simulink model "schemaABlocchi_2023b"  (R2023b)
settings: Solver=ode45  StartTime=0.0  StopTime=12  MaxStep=1e-3  RelTol=1e-3  EnableMultiTasking=on
PreLoadFcn:
  | clear %%clear workspace
  | 
  | %--------------------
  | %SYSTEM'S PARAMETERS [parametri del sistema]:
  | %--------------------
  | 
  | M = 0.5         %cart mass [massa del carrello]
  | m = 0.1         %sphere mass [massa estremità del asta]
  | g = 9,80665     %gravity acceleration [accelerazione gravità]
  | L = 0.3         %rod length [lunghezza asta]
  | 
  | %--------------------
  | %STATE EQUATIONS [matrici di stato]:
  | %--------------------
  | A = [ 0 1  0             0;
  |       0 0  -(m*g)/M      0;
  |       0 0  0             1;
  |       0 0  (M+m)*g/(L*M) 0]
  | B = [ 0 ;
  |       1/M;
  |       0;
  |       -1/(L*M)]
  | C = [1 0 0 0;
  |      0 0 1 0]
  | 
  | D = zeros(size(C,1),size(B,2)) % [sistema strettamente proprio]
  | 
  | dimx = size(A,1) % A dimention [dimensione matrice quadrata "A"]
  | dimu = size(B,2) % B column [numero colonne matrice "B"]
  | dimy = size(C,1) % C row [numero righe matrice "C"]
  | 
  | %--------------------
  | %INITIAL CONDITIONS SYSTEM(state) AND OBSERVER(estimated state) [condizioni iniziali sistema e osservatore]
  | %--------------------
  | 
  | x0 = [.5;               %initial cart position (meter) [posizione iniziale del carrello]
  |       .1;               %initial cart speed (meter/s) [velocità iniziale del carrello]
  |       20;       %initial rod angle ("degree" *pi/180 = radiants) [angolo iniziale dell'asta]
  |       .1]      %initial rod angular speed ("degree/seconds" *pi/180 = radiants/seconds) [velocità angolare asta]
  | 
  | % x0 = [0 0 0 0]';      % [punto di equilibrio]
libraries: vrlib x3, sldrtlib x1
settings Model: Creator=giassai  LastModifiedBy=simone
settings SolverCC: ZeroCrossAlgorithm=Non-adaptive  AlgebraicLoopSolver=TrustRegion
settings DataIOCC: LimitDataPoints=on  SaveFormat=Array  SignalLoggingSaveFormat=ModelDataLogs  ReturnWorkspaceOutputs=off
settings OptimizationCC: ExpressionDepthLimit=2147483647  InitFltsAndDblsToZero=on  LifeSpan=inf
settings DebuggingCC: UnderspecifiedInitializationDetection=Classic  MergeDetectMultiDrivingBlocksExec=none  SolverPrmCheckMsg=warning  FcnCallInpInsideContextMsg=warning  UnconnectedInputMsg=warning  UnconnectedOutputMsg=warning  UnconnectedLineMsg=warning  StateNameClashWarn=warning  SFUnexpectedBacktrackingDiag=warning  SFNoUnconditionalDefaultTransitionDiag=warning  SFExecutionAtInitializationDiag=none  ArithmeticOperatorsInVariantConditions=warning
settings HardwareCC: ProdBitPerPointer=32  ProdBitPerSizeT=32  ProdBitPerPtrDiffT=32  ProdLargestAtomicFloat=None  ProdIntDivRoundTo=Undefined  ProdEndianess=Unspecified  ProdWordSize=32  ProdHWDeviceType=32-bit Generic
settings ModelReferenceCC: PropagateSignalLabelsOutOfModel=off
settings CodeAppCC: StateflowObjectComments=on
settings GRTTargetCC: TargetLangStandard=C89/C90 (ANSI)  CombineOutputUpdateFcns=off  GRTInterface=on
settings ConfigComp: CovMetricSettings=dw  CovSaveCumulativeToWorkspaceVar=on  CovSaveSingleToWorkspaceVar=on

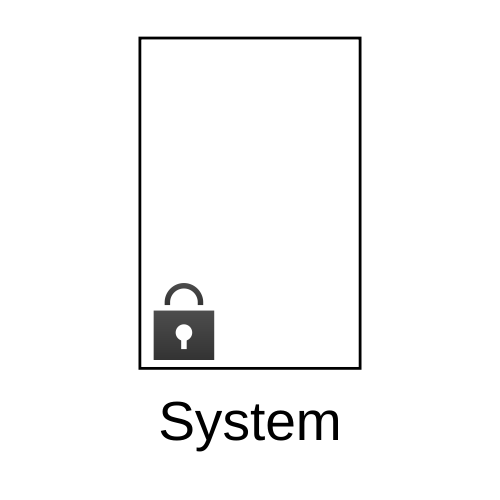
[thumbnail: Simulink's stored preview of the top-level diagram]
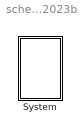
== system schemaABlocchi_2023b ==
  System : Subsystem

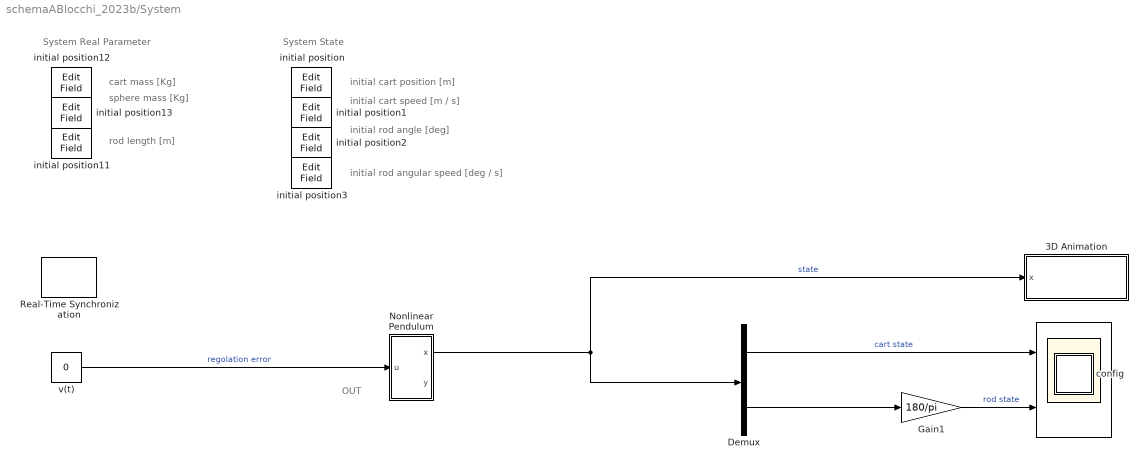
== system schemaABlocchi_2023b/System ==
  note: OUT
  note: System Real Parameter
  note: sphere mass [Kg]
  note: rod length [m]
  note: cart mass [Kg]
  note: initial rod angular speed [deg / s]
  note: initial rod angle [deg]
  note: initial cart speed [m / s]
  note: initial cart position [m]
  note: System State
  " " : Scope  NumInputPorts=2
  3D Animation : Subsystem
  Demux : Demux  Outputs=2
  Gain1 : Gain  Gain=180/pi
  Nonlinear Pendulum : Subsystem
  Real-Time Synchronization : sldrtlib/Real-Time Synchronization  SampleTime=0.01  MaxMissedTicks=500  ShowMissedTicks=off  YieldWhenWaiting=off
  config : Subsystem
  initial position{,1..3,11..13} (7 alike) : EditField  LabelPosition=Hide  ShowInitialText=on  Alignment=Center
  v(t) : Constant  Value=0
  wires:
  v(t)/1 -> Nonlinear Pendulum/1(u)  "regolation error"
  Demux/2 -> Gain1/1
  Nonlinear Pendulum/1(x) -> 3D Animation/1(x), Demux/1  "state"
  Gain1/1 -> " "/2  "rod state"
  Demux/1 -> " "/1  "cart state"

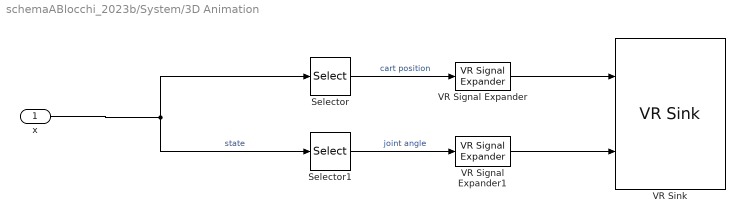
== system schemaABlocchi_2023b/System/3D Animation ==
  x : Inport
  Selector : Selector  InputPortWidth=4  IndexOptions=Index vector (dialog)  Indices=[1]  OutputSizes=1  RuntimeRangeChecks=on
  Selector1 : Selector  InputPortWidth=4  IndexOptions=Index vector (dialog)  Indices=[3]  OutputSizes=1  RuntimeRangeChecks=on
  VR Signal Expander : vrlib/VR Signal Expander  outwidth=3  outidx=[1]
  VR Signal Expander1 : vrlib/VR Signal Expander  outwidth=4  outidx=[4]
  VR Sink : vrlib/VR Sink  InstantiateOnLoad=on  SampleTime=0.1  ViewEnable=on  RemoteChange=off  RemoteView=off  FieldsWritten=cart.translation.3.1.1.double#joint.rotation.4.1.1.double  WorldFileName=modello3D.wrl  AutoView=on  VideoDimensions=[]  AllowVariableSize=off  FigureProperties="{'Position', 'Name', 'Viewpoint', 'CameraBound', 'CameraDirection', 'CameraPosition', 'CameraUpVector', 'ZoomFactor', 'Antialiasing', 'Headlight', 'Lighting', 'Sound', 'StatusBar', 'Stereo3D', 'Stereo3DCameraOffset', 'Stereo3DHIT', 'ToolBar', 'Textures', 'Transparency', 'Triad', 'Wireframe', 'NavZones', 'NavMode', 'NavSpeed', 'CaptureFileFormat', 'CaptureFileName', 'Record2DCompressMethod', 'Record2DCompressQuality', 'Record2D', 'Record2DFileName', 'Record2DFPS', 'NavPanel'; [1.3670000000000000e+03   1.2500000000000000e+02   1.3890000000000000e+03   9.0400000000000000e+02], '', 'frontal view', 'on', [0.0000000000000000e+00   0.0000000000000000e+00  -1.0000000000000000e+00], [0.0000000000000000e+00   0.0000000000000000e+00   0.0000000000000000e+00], [0.0000000000000000e+00   1.0000000000000000e+00   0.0000000000000000e+00], [1.0000000000000000e+00], 'on', 'on', 'on', 'on', 'on', 'off', [1.0000000149011612e-01], [0.0000000000000000e+00], 'on', 'on', 'on', 'none', 'off', 'off', 'fly', 'normal', 'tif', '%f_anim_%n.tif', 'auto', [7.5000000000000000e+01], 'off', '%f_anim_%n.avi', 'auto', 'halfbar'}"
  wires:
  Selector/1 -> VR Signal Expander/1  "cart position"
  x/1 -> Selector1/1, Selector/1  "state"
  Selector1/1 -> VR Signal Expander1/1  "joint angle"
  VR Signal Expander1/1 -> VR Sink/2
  VR Signal Expander/1 -> VR Sink/1

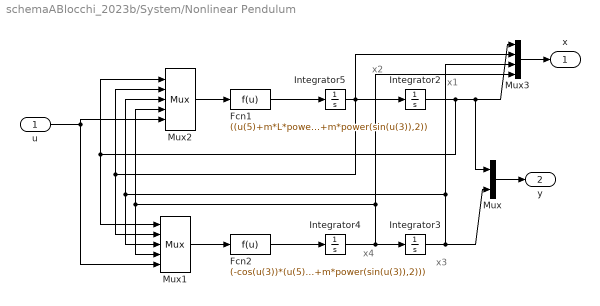
== system schemaABlocchi_2023b/System/Nonlinear Pendulum ==
  note: x1
  note: x2
  note: x3
  note: x4
  u : Inport
  Fcn1 : Fcn  Expr=((u(5)+m*L*power(sin(u(3)),1)*power(u(4),2))-m*sin(u(3))*cos(u(3))*g)/(M+m*power(sin(u(3)),2))
  Fcn2 : Fcn  Expr=(-cos(u(3))*(u(5)+m*L*power(sin(u(3)),1)*power(u(4),2))+(M+m)*g*sin(u(3)))/(L*(M+m*power(sin(u(3)),2)))
  Integrator2 : Integrator  InitialCondition=x0(1)
  Integrator3 : Integrator  InitialCondition=x0(3)*pi/180
  Integrator4 : Integrator  InitialCondition=x0(4)*pi/180
  Integrator5 : Integrator  InitialCondition=x0(2)
  Mux : Mux  Inputs=2
  Mux1 : Mux  Inputs=5
  Mux2 : Mux  Inputs=5
  Mux3 : Mux
  x : Outport
  y : Outport  Port=2
  wires:
  Integrator2/1 -> Mux/1, Mux3/1, Mux2/1, Mux1/1
  Fcn2/1 -> Integrator4/1
  Mux1/1 -> Fcn2/1
  Mux2/1 -> Fcn1/1
  Fcn1/1 -> Integrator5/1
  Integrator5/1 -> Integrator2/1, Mux1/2, Mux2/2, Mux3/2
  Integrator4/1 -> Integrator3/1, Mux2/4, Mux1/4, Mux3/4
  Integrator3/1 -> Mux/2, Mux2/3, Mux1/3, Mux3/3
  u/1 -> Mux2/5, Mux1/5
  Mux/1 -> y/1
  Mux3/1 -> x/1

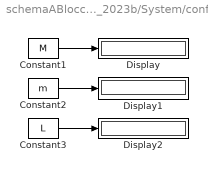
== system schemaABlocchi_2023b/System/config ==
  Constant1 : Constant  Value=M
  Constant2 : Constant  Value=m
  Constant3 : Constant  Value=L
  Display : Display
  Display1 : Display
  Display2 : Display
  wires:
  Constant2/1 -> Display1/1
  Constant3/1 -> Display2/1
  Constant1/1 -> Display/1
